simulink model "sistema"  (R2018b)
settings: Solver=VariableStepAuto  StartTime=0.0  StopTime=10.0  RelTol=1e-3
settings Model: Creator=Clesio  LastModifiedBy=Clesio

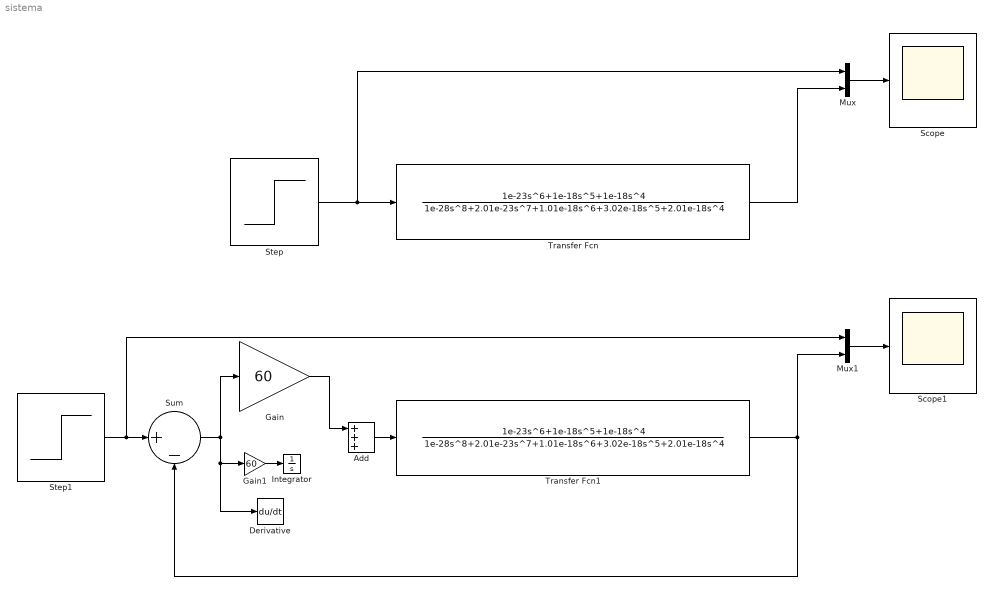
== system sistema ==
  Add : Sum  Inputs=+++
  Derivative : Derivative  CoefficientInTFapproximation=20
  Gain : Gain  Gain=60
  Gain1 : Gain  Gain=60
  Integrator : Integrator
  Mux : Mux  Inputs=2
  Mux1 : Mux  Inputs=2
  Scope : Scope
  Scope1 : Scope
  Step : Step  After=5  SampleTime=0
  Step1 : Step  After=.1  SampleTime=0
  Sum : Sum  Inputs=|+-
  Transfer Fcn : TransferFcn  Numerator=[1e-23 1e-18 1e-18 0 0 0 0]  Denominator="[1e-28 2.01e-23 1.01e-18 3.02e-18 2.01e-18  0 0 0 0]"
  Transfer Fcn1 : TransferFcn  Numerator=[1e-23 1e-18 1e-18 0 0 0 0]  Denominator="[1e-28 2.01e-23 1.01e-18 3.02e-18 2.01e-18  0 0 0 0]"
  wires:
  Step/1 -> Mux/1, Transfer Fcn/1
  Mux/1 -> Scope/1
  Transfer Fcn/1 -> Mux/2
  Sum/1 -> Derivative/1, Gain1/1, Gain/1
  Step1/1 -> Mux1/1, Sum/1
  Mux1/1 -> Scope1/1
  Transfer Fcn1/1 -> Sum/2, Mux1/2
  Add/1 -> Transfer Fcn1/1
  Gain/1 -> Add/1
  Gain1/1 -> Integrator/1
